simulink model "correcteur"  (R2018b)
settings: Solver=VariableStepAuto  StartTime=0.0  StopTime=10.0  RelTol=1e-3
settings Model: Creator=xpess  LastModifiedBy=xpess

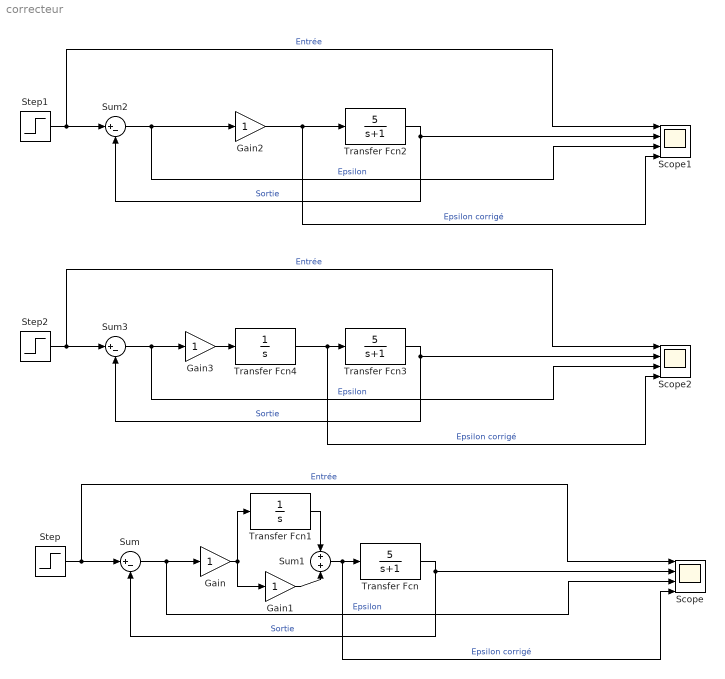
== system correcteur ==
  Gain{,1..3} (4 alike) : Gain
  Scope : Scope  NumInputPorts=4
  Scope1 : Scope  NumInputPorts=4
  Scope2 : Scope  NumInputPorts=4
  Step : Step  Time=0  SampleTime=0
  Step1 : Step  Time=0  SampleTime=0
  Step2 : Step  Time=0  SampleTime=0
  Sum : Sum  Inputs=|+-
  Sum1 : Sum  Inputs=+|+
  Sum2 : Sum  Inputs=|+-
  Sum3 : Sum  Inputs=|+-
  Transfer Fcn : TransferFcn  Numerator=[5]  Denominator=[1 1]
  Transfer Fcn1 : TransferFcn  Denominator=[1 0]
  Transfer Fcn2 : TransferFcn  Numerator=[5]  Denominator=[1 1]
  Transfer Fcn3 : TransferFcn  Numerator=[5]  Denominator=[1 1]
  Transfer Fcn4 : TransferFcn  Denominator=[1 0]
  wires:
  Transfer Fcn/1 -> Scope/2, Sum/2  "Sortie"
  Step/1 -> Scope/1, Sum/1  "Entrée"
  Sum1/1 -> Scope/4, Transfer Fcn/1  "Epsilon corrigé"
  Sum/1 -> Scope/3, Gain/1  "Epsilon"
  Gain/1 -> Gain1/1, Transfer Fcn1/1
  Transfer Fcn1/1 -> Sum1/1
  Gain1/1 -> Sum1/2
  Sum2/1 -> Gain2/1, Scope1/3  "Epsilon"
  Gain2/1 -> Transfer Fcn2/1, Scope1/4  "Epsilon corrigé"
  Step1/1 -> Sum2/1, Scope1/1  "Entrée"
  Transfer Fcn2/1 -> Sum2/2, Scope1/2  "Sortie"
  Transfer Fcn3/1 -> Scope2/2, Sum3/2  "Sortie"
  Gain3/1 -> Transfer Fcn4/1
  Sum3/1 -> Scope2/3, Gain3/1  "Epsilon"
  Transfer Fcn4/1 -> Scope2/4, Transfer Fcn3/1  "Epsilon corrigé"
  Step2/1 -> Scope2/1, Sum3/1  "Entrée"
